simulink library "Wound_Rotor_Starter"  (R2024a)
settings: Solver=VariableStepAuto  StartTime=0.0  StopTime=10.0  RelTol=1e-3
libraries: spsSeriesRLCBranchLib x9, spsThreePhaseBreakerLib x4
settings Model: Creator=gshma  LastModifiedBy=gshma

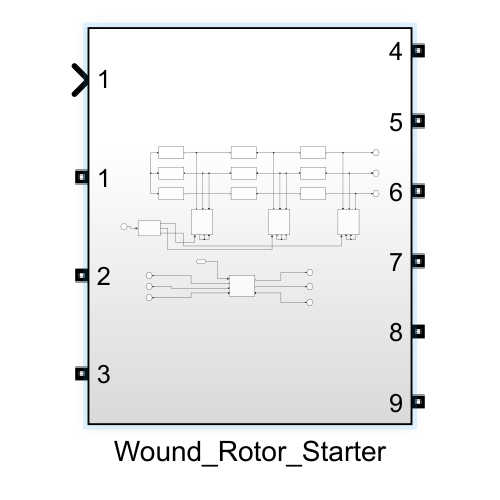
[thumbnail: Simulink's stored preview of the top-level diagram]
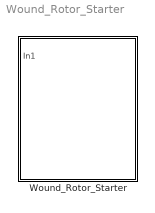
== system Wound_Rotor_Starter ==
  Wound_Rotor_Starter : Subsystem

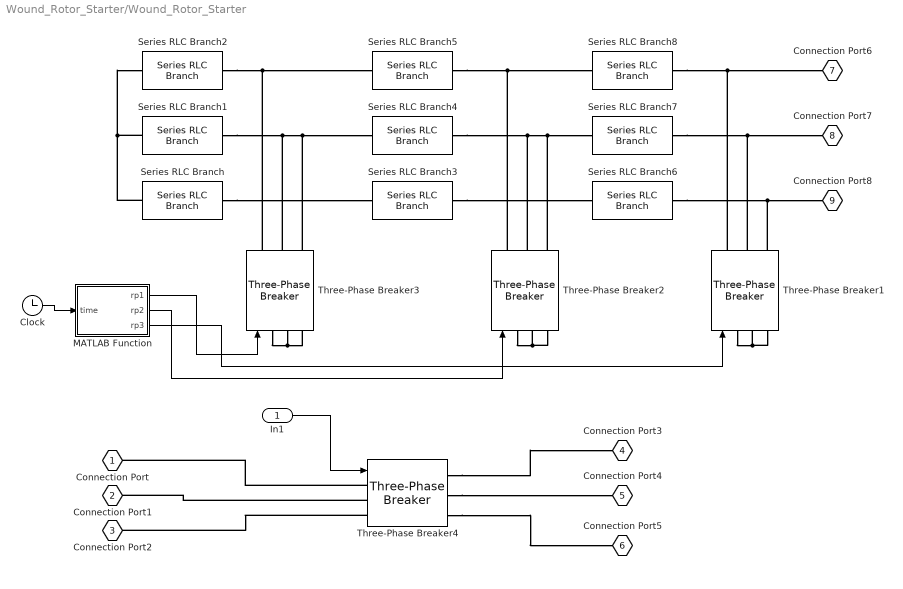
== system Wound_Rotor_Starter/Wound_Rotor_Starter ==
  In1 : Inport
  Clock : Clock
  MATLAB Function : MATLAB Function  TreatAsAtomicUnit=on
  Series RLC Branch{,1..8} (9 alike) : spsSeriesRLCBranchLib/Series RLC Branch  LConnTagsString=__new0  RConnTagsString=__new0  BranchType=R  Resistance=4.8  Inductance=1e-3  SetiL0=off  InitialCurrent=0  Capacitance=1e-6  Setx0=off  InitialVoltage=0  Measurements=None
  Three-Phase Breaker1 : spsThreePhaseBreakerLib/Three-Phase Breaker  InitialState=open  SwitchA=on  SwitchB=on  SwitchC=on  SwitchTimes="[1/60  5/60]"  External=on  BreakerResistance=0.01  SnubberResistance=1e6  SnubberCapacitance=inf  Measurements=None
  Three-Phase Breaker2 : spsThreePhaseBreakerLib/Three-Phase Breaker  InitialState=open  SwitchA=on  SwitchB=on  SwitchC=on  SwitchTimes="[1/60  5/60]"  External=on  BreakerResistance=0.01  SnubberResistance=1e6  SnubberCapacitance=inf  Measurements=None
  Three-Phase Breaker3 : spsThreePhaseBreakerLib/Three-Phase Breaker  InitialState=open  SwitchA=on  SwitchB=on  SwitchC=on  SwitchTimes="[1/60  5/60]"  External=on  BreakerResistance=0.01  SnubberResistance=1e6  SnubberCapacitance=inf  Measurements=None
  Three-Phase Breaker4 : spsThreePhaseBreakerLib/Three-Phase Breaker  InitialState=closed  SwitchA=on  SwitchB=on  SwitchC=on  SwitchTimes="[1/60  5/60]"  External=on  BreakerResistance=0.01  SnubberResistance=1e6  SnubberCapacitance=inf  Measurements=None
  Connection Port : PMIOPort  Tag=simrfV2util1/Connection Port  Side=Left
  Connection Port1 : PMIOPort  Tag=simrfV2util1/Connection Port  Port=2  Side=Left
  Connection Port2 : PMIOPort  Tag=simrfV2util1/Connection Port  Port=3  Side=Left
  Connection Port3 : PMIOPort  Tag=simrfV2util1/Connection Port  Port=4  Side=Right
  Connection Port4 : PMIOPort  Tag=simrfV2util1/Connection Port  Port=5  Side=Right
  Connection Port5 : PMIOPort  Tag=simrfV2util1/Connection Port  Port=6  Side=Right
  Connection Port6 : PMIOPort  Tag=simrfV2util1/Connection Port  Port=7  Side=Right
  Connection Port7 : PMIOPort  Tag=simrfV2util1/Connection Port  Port=8  Side=Right
  Connection Port8 : PMIOPort  Tag=simrfV2util1/Connection Port  Port=9  Side=Right
  wires:
  In1/1 -> Three-Phase Breaker4/1
  Clock/1 -> MATLAB Function/1(time)
  MATLAB Function/1(rp1) -> Three-Phase Breaker3/1
  MATLAB Function/2(rp2) -> Three-Phase Breaker2/1
  MATLAB Function/3(rp3) -> Three-Phase Breaker1/1
  connections:
  Series RLC Branch2/LConn1 -- Three-Phase Breaker3/RConn1 -- Series RLC Branch5/RConn1
  Series RLC Branch1/LConn1 -- Three-Phase Breaker3/RConn2 -- Three-Phase Breaker3/RConn3 -- Series RLC Branch4/RConn1
  Series RLC Branch/LConn1 -- Series RLC Branch3/RConn1
  Series RLC Branch5/LConn1 -- Three-Phase Breaker2/RConn1 -- Series RLC Branch8/RConn1
  Series RLC Branch4/LConn1 -- Three-Phase Breaker2/RConn2 -- Series RLC Branch7/RConn1 -- Three-Phase Breaker2/RConn3
  Series RLC Branch3/LConn1 -- Series RLC Branch6/RConn1
  Series RLC Branch8/LConn1 -- Three-Phase Breaker1/RConn1 -- Connection Port6/RConn1
  Series RLC Branch7/LConn1 -- Three-Phase Breaker1/RConn2 -- Connection Port7/RConn1
  Series RLC Branch6/LConn1 -- Three-Phase Breaker1/RConn3 -- Connection Port8/RConn1
  Series RLC Branch1/RConn1 -- Series RLC Branch/RConn1 -- Series RLC Branch2/RConn1
  Three-Phase Breaker4/LConn1 -- Connection Port/RConn1
  Three-Phase Breaker4/LConn2 -- Connection Port1/RConn1
  Three-Phase Breaker4/LConn3 -- Connection Port2/RConn1
  Three-Phase Breaker4/RConn1 -- Connection Port3/RConn1
  Three-Phase Breaker4/RConn2 -- Connection Port4/RConn1
  Three-Phase Breaker4/RConn3 -- Connection Port5/RConn1
  Three-Phase Breaker3/LConn2 -- Three-Phase Breaker3/LConn3 -- Three-Phase Breaker3/LConn1
  Three-Phase Breaker2/LConn1 -- Three-Phase Breaker2/LConn3 -- Three-Phase Breaker2/LConn2
  Three-Phase Breaker1/LConn1 -- Three-Phase Breaker1/LConn3 -- Three-Phase Breaker1/LConn2

== matlab function Wound_Rotor_Starter/MATLAB Function ==
  data: time input; rp1 output; rp2 output; rp3 output
function [rp1,rp2,rp3] = fcn(time)
    if time<2
        rp1 = false;
        rp2 = false;
        rp3 = false;
    elseif time>=2 && time<4
        rp1 = true;
        rp2 = false;
        rp3 = false;
    elseif time>=4 && time<5
        rp1 = true;
        rp2 = true;
        rp3 = false;
    else
        rp1 = true;
        rp2 = true;
        rp3 = true;
    end
end
